simulink model "Simple_Model"  (R2023a)
settings: Solver=VariableStepAuto  StartTime=0.0  StopTime=1000  RelTol=1e-3
libraries: SignalEditorBlockLib x3, dspsigops x1
settings Model: Creator=levir  LastModifiedBy=levir

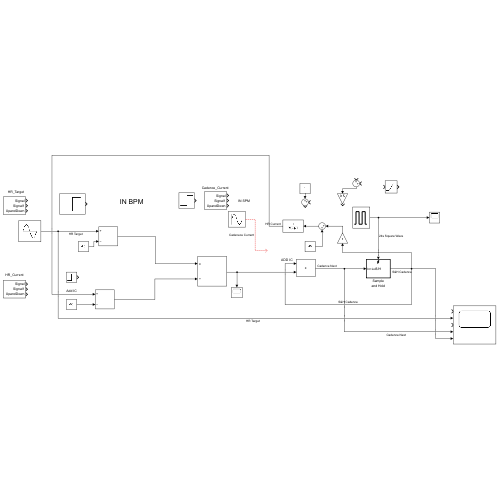
[thumbnail: Simulink's stored preview of the top-level diagram]
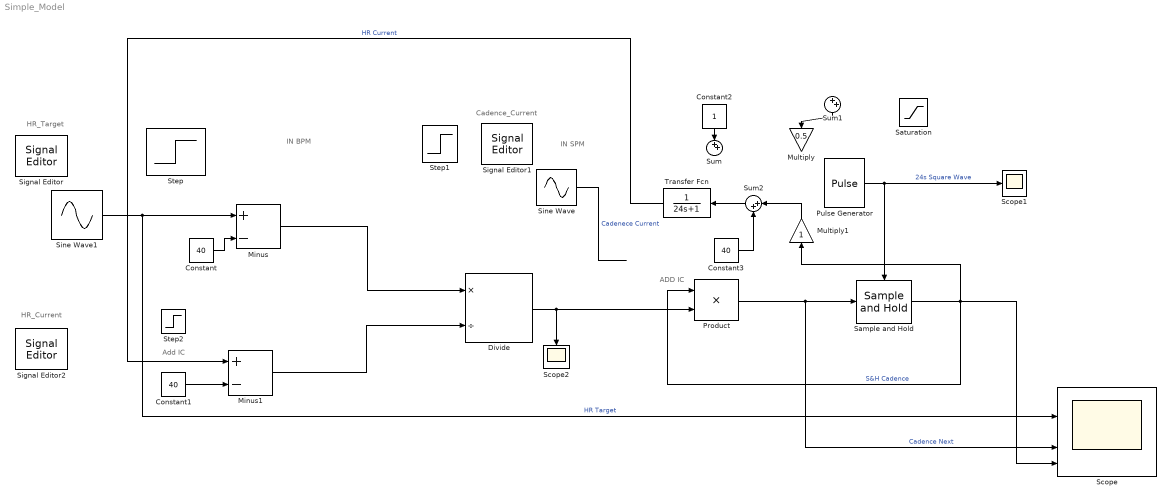
== system Simple_Model ==
  note: ADD IC
  note: Add IC
  note: IN BPM
  note: IN SPM
  note: Cadence_Current
  note: HR_Current
  note: HR_Target
  Constant : Constant  Value=40
  Constant1 : Constant  Value=40
  Constant2 : Constant
  Constant3 : Constant  Value=40
  Divide : Product  Inputs=*/
  Minus : Sum  Inputs=+-
  Minus1 : Sum  Inputs=+-
  Multiply : Gain  Gain=0.5
  Multiply1 : Gain
  Product : Product
  Pulse Generator : DiscretePulseGenerator  PulseType=Time based  Period=15  PulseWidth=10
  Sample and Hold : dspsigops/Sample and Hold  trig=Rising edge  initCond=0  latchinput=on
  Saturation : Saturate  UpperLimit=200  LowerLimit=80
  Scope : Scope  NumInputPorts=5
  Scope1 : Scope
  Scope2 : Scope
  Signal Editor : SignalEditorBlockLib/Signal Editor  FileName=C:\Users\levir\OneDrive\Documents\MATLAB\Thesis\testingWave.mat  ActiveScenario=Scenario  ActiveSignal=Signal  IsBus=off  OutputBusObjectStr=Bus: BusObject  SampleTime=0  Interpolate=off  ZeroCross=off  OutputAfterFinalValue=Setting to zero  Unit=inherit  PreserveSignalName=on  ApplySigPropsToAllScenarios=on
  Signal Editor1 : SignalEditorBlockLib/Signal Editor  FileName=C:\Users\levir\OneDrive\Documents\MATLAB\Thesis\testingWave.mat  ActiveScenario=Scenario  ActiveSignal=Signal  IsBus=off  OutputBusObjectStr=Bus: BusObject  SampleTime=0  Interpolate=off  ZeroCross=off  OutputAfterFinalValue=Setting to zero  Unit=inherit  PreserveSignalName=on  ApplySigPropsToAllScenarios=on
  Signal Editor2 : SignalEditorBlockLib/Signal Editor  FileName=C:\Users\levir\OneDrive\Documents\MATLAB\Thesis\testingWave.mat  ActiveScenario=Scenario  ActiveSignal=Signal  IsBus=off  OutputBusObjectStr=Bus: BusObject  SampleTime=0  Interpolate=off  ZeroCross=off  OutputAfterFinalValue=Setting to zero  Unit=inherit  PreserveSignalName=on  ApplySigPropsToAllScenarios=on
  Sine Wave : Sin  Amplitude=20  Bias=120  Frequency=0.01  SampleTime=0
  Sine Wave1 : Sin  Amplitude=20  Bias=120  Frequency=0.01  SampleTime=0
  Step : Step  After=140  SampleTime=0
  Step1 : Step  After=100  SampleTime=0
  Step2 : Step  SampleTime=0
  Sum : Sum  Inputs=|++
  Sum1 : Sum  Inputs=|++
  Sum2 : Sum  Inputs=|++
  Transfer Fcn : TransferFcn  Denominator=[24 1]
  wires:
  Constant/1 -> Minus/2
  Minus/1 -> Divide/1
  Constant1/1 -> Minus1/2
  Minus1/1 -> Divide/2
  Divide/1 -> Product/2, Scope2/1
  Product/1 -> Scope/4, Sample and Hold/1  "Cadence Next"
  Pulse Generator/1 -> Scope1/1, Sample and Hold/Trigger  "24s Square Wave"
  Sine Wave1/1 -> Minus/1, Scope/2  "HR Target"
  Sample and Hold/1 -> Product/1, Scope/5, Multiply1/1  "S&H Cadence"
  Constant2/1 -> Sum/1
  Sum1/1 -> Multiply/1
  Constant3/1 -> Sum2/2
  Multiply1/1 -> Sum2/1
  Sum2/1 -> Transfer Fcn/1
  Sine Wave/1 -> ?  "Cadenece Current"
  Transfer Fcn/1 -> Minus1/1  "HR Current"
